simulink model "ans16_1"  (R2019a)
settings: Solver=VariableStepAuto  StartTime=0.0  StopTime=10.0  RelTol=1e-3
undefined symbols (not defined in the file or in its folder): KD, KI, KP, qr_i
settings Model: Creator=andylei  LastModifiedBy=matth
settings DataIOCC: SaveFormat=StructureWithTime  ReturnWorkspaceOutputs=off
settings DebuggingCC: ArithmeticOperatorsInVariantConditions=warning

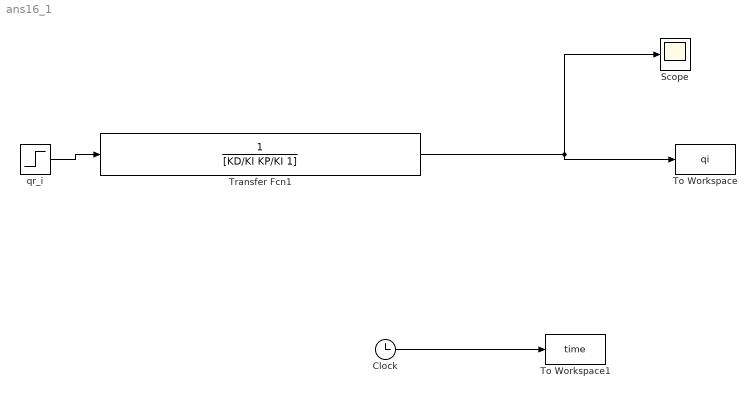
== system ans16_1 ==
  Clock : Clock
  Scope : Scope
  To Workspace : ToWorkspace  VariableName=qi  SampleTime=-1
  To Workspace1 : ToWorkspace  VariableName=time  SampleTime=-1
  Transfer Fcn1 : TransferFcn  Denominator=[KD/KI KP/KI 1]
  qr_i : Step  Before=qr_i  After=qr_i  SampleTime=0
  wires:
  qr_i/1 -> Transfer Fcn1/1
  Transfer Fcn1/1 -> To Workspace/1, Scope/1
  Clock/1 -> To Workspace1/1
